simulink model "modele_dyskretne"  (R2021a)
settings: Solver=VariableStepAuto  StartTime=0.0  StopTime=70  RelTol=1e-3
values from neighbouring files (symbols this model uses):
  a1 = 0.32    [Wartosci_w_zadaniu.m]    (also in zad_4.m)
  a2 = 0.45    [Wartosci_w_zadaniu.m]    (also in zad_4.m)
  a3 = -0.29    [Wartosci_w_zadaniu.m]    (also in zad_4.m)
  a4 = -0.1    [Wartosci_w_zadaniu.m]    (also in zad_4.m)
  K = 2    [Wartosci_w_zadaniu.m]    (also in zad_4.m)
  T = 1.5    [zad_4.m]
  T1 = 5    [Wartosci_w_zadaniu.m]    (also in zad_4.m)
  T2 = 8    [Wartosci_w_zadaniu.m]    (also in zad_4.m)
  u_0 = -0.85    [zad_5_i_6.m]
settings Model: Creator=ADMIN  LastModifiedBy=ADMIN

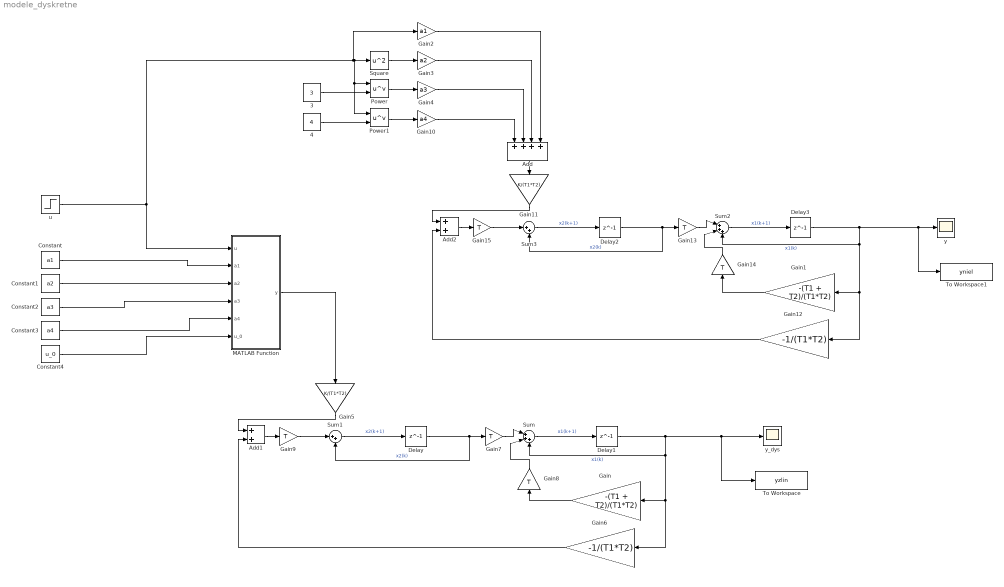
== system modele_dyskretne ==
  " 3" : Constant  Value=3
  4 : Constant  Value=4
  Add : Sum  Inputs=++++
  Add1 : Sum
  Add2 : Sum
  Constant : Constant  Value=a1
  Constant1 : Constant  Value=a2
  Constant2 : Constant  Value=a3
  Constant3 : Constant  Value=a4
  Constant4 : Constant  Value=u_0
  Delay{,1..3} (4 alike) : Delay  DelayLength=1  InitialCondition=0  SampleTime=T
  Gain : Gain  Gain=-(T1 + T2)/(T1*T2)
  Gain1 : Gain  Gain=-(T1 + T2)/(T1*T2)
  Gain10 : Gain  Gain=a4
  Gain11 : Gain  Gain=K/(T1*T2)
  Gain12 : Gain  Gain=-1/(T1*T2)
  Gain{7..9,13..15} (6 alike) : Gain  Gain=T
  Gain2 : Gain  Gain=a1
  Gain3 : Gain  Gain=a2
  Gain4 : Gain  Gain=a3
  Gain5 : Gain  Gain=K/(T1*T2)
  Gain6 : Gain  Gain=-1/(T1*T2)
  MATLAB Function : MATLAB Function  TreatAsAtomicUnit=on
  Power : Math  Operator=pow  SaturateOnIntegerOverflow=on
  Power1 : Math  Operator=pow  SaturateOnIntegerOverflow=on
  Square : Math  Operator=square  SaturateOnIntegerOverflow=on
  Sum : Sum  Inputs=|+++
  Sum1 : Sum  Inputs=|++
  Sum2 : Sum  Inputs=|+++
  Sum3 : Sum  Inputs=|++
  To Workspace : ToWorkspace  VariableName=yzlin  SaveFormat=Structure With Time  SampleTime=T
  To Workspace1 : ToWorkspace  VariableName=yniel  SaveFormat=Structure With Time  SampleTime=T
  u : Step  SampleTime=0
  y : Scope
  y_dys : Scope
  wires:
  Constant2/1 -> MATLAB Function/4(a3)
  Gain8/1 -> Sum/2
  Gain9/1 -> Sum1/1
  Delay1/1 -> Sum/3, Gain6/1, Gain/1, To Workspace/1, y_dys/1  "x1(k)"
  Gain5/1 -> Add1/1
  Gain6/1 -> Add1/2
  Gain/1 -> Gain8/1
  Delay/1 -> Sum1/2, Gain7/1  "x2(k)"
  Sum1/1 -> Delay/1  "x2(k+1)"
  Add1/1 -> Gain9/1
  Gain7/1 -> Sum/1
  Constant4/1 -> MATLAB Function/6(u_0)
  MATLAB Function/1(y) -> Gain5/1
  Sum/1 -> Delay1/1  "x1(k+1)"
  Constant/1 -> MATLAB Function/2(a1)
  Constant3/1 -> MATLAB Function/5(a4)
  Constant1/1 -> MATLAB Function/3(a2)
  " 3"/1 -> Power/2
  u/1 -> MATLAB Function/1(u), Gain2/1, Power1/1, Power/1, Square/1
  4/1 -> Power1/2
  Sum3/1 -> Delay2/1  "x2(k+1)"
  Square/1 -> Gain3/1
  Gain4/1 -> Add/2
  Gain11/1 -> Add2/1
  Power/1 -> Gain4/1
  Gain3/1 -> Add/3
  Gain15/1 -> Sum3/1
  Add2/1 -> Gain15/1
  Power1/1 -> Gain10/1
  Gain10/1 -> Add/1
  Add/1 -> Gain11/1
  Delay3/1 -> Sum2/3, Gain12/1, Gain1/1, To Workspace1/1, y/1  "x1(k)"
  Gain2/1 -> Add/4
  Gain13/1 -> Sum2/1
  Gain12/1 -> Add2/2
  Delay2/1 -> Sum3/2, Gain13/1  "x2(k)"
  Gain1/1 -> Gain14/1
  Gain14/1 -> Sum2/2
  Sum2/1 -> Delay3/1  "x1(k+1)"

== matlab function modele_dyskretne/MATLAB Function ==
  data: u input; y output; a1 input; a2 input; a3 input; a4 input; u_0 input
function y = fcn(u,a1,a2,a3,a4,u_0)
y = a1* u + a2*((u_0)^2 + 2*u_0*(u-u_0)) + a3*((u_0)^3 + 3*(u_0^2)*(u-u_0)) + a4*((u_0)^4 + 4*(u_0^3)*(u-u_0));
end
